simulink model "cart_pole_plant"  (R2015b)
settings: Solver=VariableStepAuto  StartTime=0.0  StopTime=10.0  RelTol=1e-3
values from neighbouring files (symbols this model uses):
  g = 9.81    [StartSim.m]
  l = 0.3    [StartSim.m]
  m = 0.2    [StartSim.m]
  M = 2    [StartSim.m]
libraries: simulink x2, aerolibconvert2 x1
settings Model: Creator=Helene  LastModifiedBy=Helene

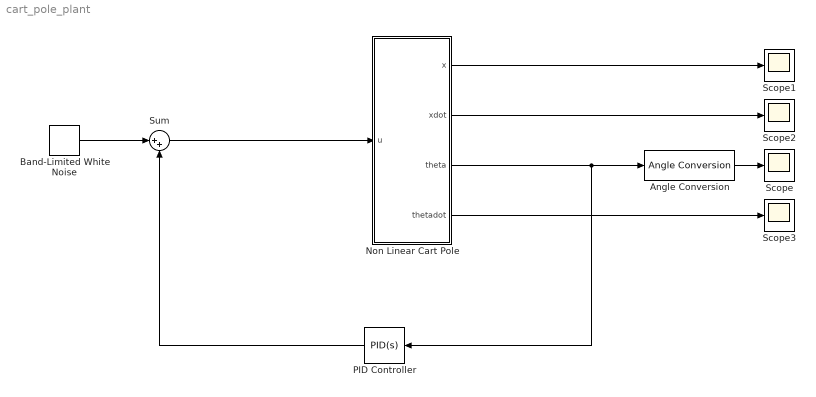
== system cart_pole_plant ==
  Angle Conversion : aerolibconvert2/Angle Conversion  IU=rad  OU=deg
  Band-Limited White Noise : simulink/Sources/Band-Limited White Noise  Cov=[4]  Ts=0.01  seed=[23341]
  Non Linear Cart Pole : Subsystem
  PID Controller : simulink/Continuous/PID Controller  Controller=PID  TimeDomain=Continuous-time  SampleTime=-1  IntegratorMethod=Forward Euler  FilterMethod=Forward Euler  Form=Parallel  UseFilter=on  ControllerParametersSource=internal  P=-78.468070295183  I=-69.9348496607617  D=-4.63399813247295  N=9.96722491148587  InitialConditionSource=internal  InitialConditionForIntegrator=0  InitialConditionForFilter=0  ExternalReset=none  LimitOutput=off  UpperSaturationLimit=inf  LowerSaturationLimit=-inf  LinearizeAsGain=on  AntiWindupMode=none  Kb=1  TrackingMode=off  Kt=1  PParamMin=[]  PParamMax=[]  IParamMin=[]  IParamMax=[]  DParamMin=[]  DParamMax=[]  NParamMin=[]  NParamMax=[]  KbParamMin=[]  KbParamMax=[]  KtParamMin=[]  KtParamMax=[]  POutMin=[]  POutMax=[]  IOutMin=[]  IOutMax=[]  DOutMin=[]  DOutMax=[]  NOutMin=[]  NOutMax=[]  KbOutMin=[]  KbOutMax=[]  KtOutMin=[]  KtOutMax=[]  IntegratorOutMin=[]  IntegratorOutMax=[]  FilterOutMin=[]  FilterOutMax=[]  SumOutMin=[]  SumOutMax=[]  SumI1OutMin=[]  SumI1OutMax=[]  SumI2OutMin=[]  SumI2OutMax=[]  SumI3OutMin=[]  SumI3OutMax=[]  SumDOutMin=[]  SumDOutMax=[]  SaturationOutMin=[]  SaturationOutMax=[]  IntegratorContinuousStateAttributes=''  IntegratorStateMustResolveToSignalObject=off  IntegratorRTWStateStorageClass=Auto  FilterContinuousStateAttributes=''  FilterStateMustResolveToSignalObject=off  FilterRTWStateStorageClass=Auto  DifferentiatorICPrevScaledInput=0  DifferentiatorOutMin=[]  DifferentiatorOutMax=[]
  Scope{,1..3} (4 alike) : Scope
  Sum : Sum  Inputs=|++
  wires:
  Non Linear Cart Pole/3(theta) -> PID Controller/1, Angle Conversion/1
  Non Linear Cart Pole/1(x) -> Scope1/1
  Non Linear Cart Pole/2(xdot) -> Scope2/1
  Non Linear Cart Pole/4(thetadot) -> Scope3/1
  Band-Limited White Noise/1 -> Sum/1
  Sum/1 -> Non Linear Cart Pole/1(u)
  PID Controller/1 -> Sum/2
  Angle Conversion/1 -> Scope/1

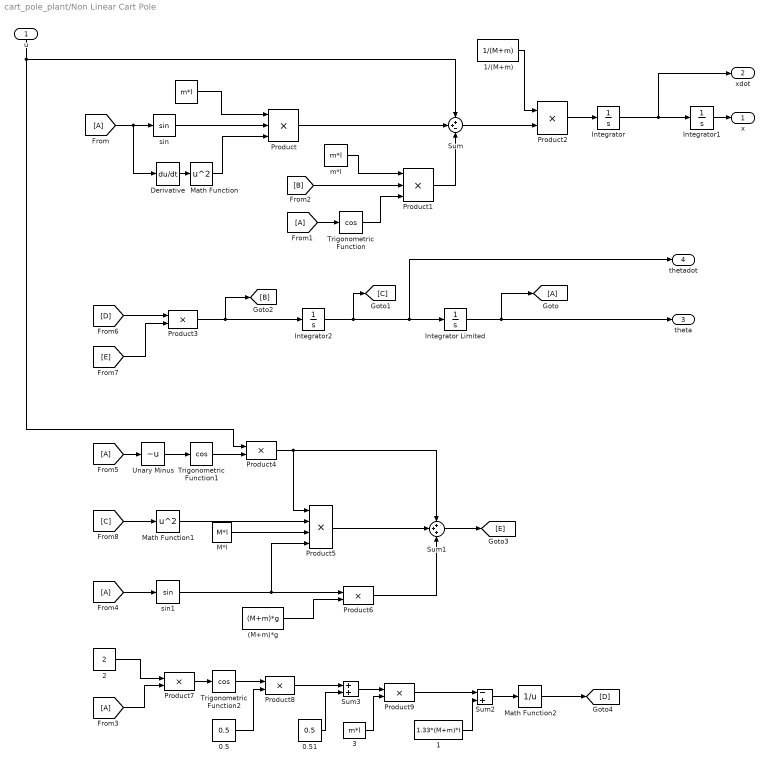
== system cart_pole_plant/Non Linear Cart Pole ==
  u : Inport
  " " : Constant  Value=m*l
  (M+m)*g : Constant  Value=(M+m)*g
  0.5 : Constant  Value=0.5
  0.51 : Constant  Value=0.5
  1 : Constant  Value=1.33*(M+m)*l
  1/(M+m) : Constant  Value=1/(M+m)
  2 : Constant  Value=2
  3 : Constant  Value=m*l
  Derivative : Derivative
  Integrator : Integrator
  Integrator Limited : Integrator  LimitOutput=on  UpperSaturationLimit=0.5*pi  LowerSaturationLimit=-0.5*pi
  Integrator1 : Integrator
  Integrator2 : Integrator
  M*l : Constant  Value=M*l
  Math Function : Math  Operator=square  SaturateOnIntegerOverflow=on
  Math Function1 : Math  Operator=square  SaturateOnIntegerOverflow=on
  Math Function2 : Math  Operator=reciprocal  SaturateOnIntegerOverflow=on
  Product : Product  Inputs=3
  Product1 : Product  Inputs=3
  Product{2..4,6..9} (7 alike) : Product
  Product5 : Product  Inputs=4
  Sum : Sum  Inputs=++-
  Sum1 : Sum  Inputs=+++
  Sum2 : Sum  Inputs=-+
  Sum3 : Sum
  Trigonometric Function : Trigonometry  Operator=cos
  Trigonometric Function1 : Trigonometry  Operator=cos
  Trigonometric Function2 : Trigonometry  Operator=cos
  Unary Minus : UnaryMinus
  m*l : Constant  Value=m*l
  sin : Trigonometry
  sin1 : Trigonometry
  x : Outport
  xdot : Outport  Port=2
  theta : Outport  Port=3
  thetadot : Outport  Port=4
  wires:
  u/1 -> Product4/1, Sum/1
  m*l/1 -> Product1/1
  Product/1 -> Sum/2
  [A] -> Trigonometric Function/1
  [A] -> Derivative/1, sin/1
  Math Function/1 -> Product/3
  [B] -> Product1/2
  Trigonometric Function/1 -> Product1/3
  sin/1 -> Product/2
  Product1/1 -> Sum/3
  Derivative/1 -> Math Function/1
  " "/1 -> Product/1
  1/(M+m)/1 -> Product2/1
  Sum/1 -> Product2/2
  Product2/1 -> Integrator/1
  Integrator/1 -> xdot/1, Integrator1/1
  Integrator1/1 -> x/1
  [D] -> Product3/1
  Product3/1 -> Integrator2/1, [B]
  Integrator2/1 -> thetadot/1, Integrator Limited/1, [C]
  Integrator Limited/1 -> [A], theta/1
  [E] -> Product3/2
  Trigonometric Function1/1 -> Product4/2
  Product4/1 -> Product5/1, Sum1/1
  Math Function1/1 -> Product5/2
  [C] -> Math Function1/1
  M*l/1 -> Product5/3
  [A] -> sin1/1
  sin1/1 -> Product5/4, Product6/1
  (M+m)*g/1 -> Product6/2
  Product5/1 -> Sum1/2
  Product6/1 -> Sum1/3
  Sum1/1 -> [E]
  2/1 -> Product7/1
  [A] -> Product7/2
  Product7/1 -> Trigonometric Function2/1
  0.5/1 -> Product8/2
  Trigonometric Function2/1 -> Product8/1
  Product8/1 -> Sum3/1
  Sum2/1 -> Math Function2/1
  Math Function2/1 -> [D]
  1/1 -> Sum2/2
  0.51/1 -> Sum3/2
  Sum3/1 -> Product9/1
  3/1 -> Product9/2
  Product9/1 -> Sum2/1
  [A] -> Unary Minus/1
  Unary Minus/1 -> Trigonometric Function1/1
